simulink model "ExRobotAndEnvironmentControllerContPI"  (Simulink 8.9)
settings: Solver=ode23s  StartTime=0.0  StopTime=1000  FixedStep=.01  RelTol=1e-3  EnableMultiTasking=on
values from neighbouring files (symbols this model uses):
  INITIAL_ROBOT_POS_THETA = 1.5*2    (= 3)    [InitRobotAndEnvironment.m]
  INITIAL_ROBOT_POS_X = 0    [InitRobotAndEnvironment.m]
  INITIAL_ROBOT_POS_Y = 0    [InitRobotAndEnvironment.m]
  INTER_WHEEL_DISTANCE = 0.12    [InitRobotAndEnvironment.m]
  ki_teta = omega*omega/alpha    (= 0.12)    [InitRobotAndEnvironment.m]
  kp_teta = 3*ksi*omega/alpha    (= 0.36)    [InitRobotAndEnvironment.m]
  MAX_SPEED = .5    (= 0.5)    [InitRobotAndEnvironment.m]
  T = 0.002    [InitRobotAndEnvironment.m]
  ts = SENSOR_SAMPLING_TIME    (= 0.001)    [InitRobotAndEnvironment.m]
  ts_anim = ANIMATION_SAMPLING_TIME    (= 0.01)    [InitRobotAndEnvironment.m]
undefined symbols (not defined in the file or in its folder): Env, Robot, RobotInit
settings Model: SuppressorTable=22 serialization::archive 11 0 6 0 0 0 11 0  Creator=alex  LastModifiedBy=dumasart  SnapshotBufferSize=200  SnapshotInterval=50
settings DataIOCC: SignalLoggingSaveFormat=Dataset
settings OptimizationCC: ExpressionDepthLimit=2147483647
settings SFSimCC: SimParseCustomCode=off

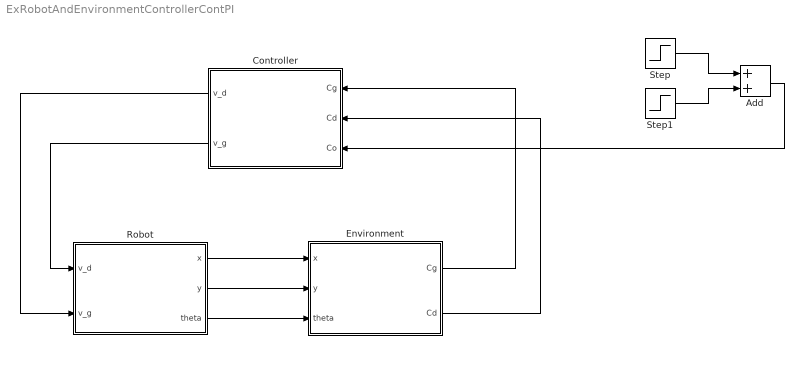
== system ExRobotAndEnvironmentControllerContPI ==
  Add : Sum
  Controller : Subsystem
  Environment : Subsystem
  Robot : Subsystem
  Step : Step  Time=2  Before=50  After=0  SampleTime=1
  Step1 : Step  Time=2.3  After=50  SampleTime=1
  wires:
  Robot/1(x) -> Environment/1(x)
  Robot/2(y) -> Environment/2(y)
  Robot/3(theta) -> Environment/3(theta)
  Environment/1(Cg) -> Controller/1(Cg)
  Environment/2(Cd) -> Controller/2(Cd)
  Controller/1(v_d) -> Robot/2(v_g)
  Controller/2(v_g) -> Robot/1(v_d)
  Step/1 -> Add/1
  Step1/1 -> Add/2
  Add/1 -> Controller/3("Co ")

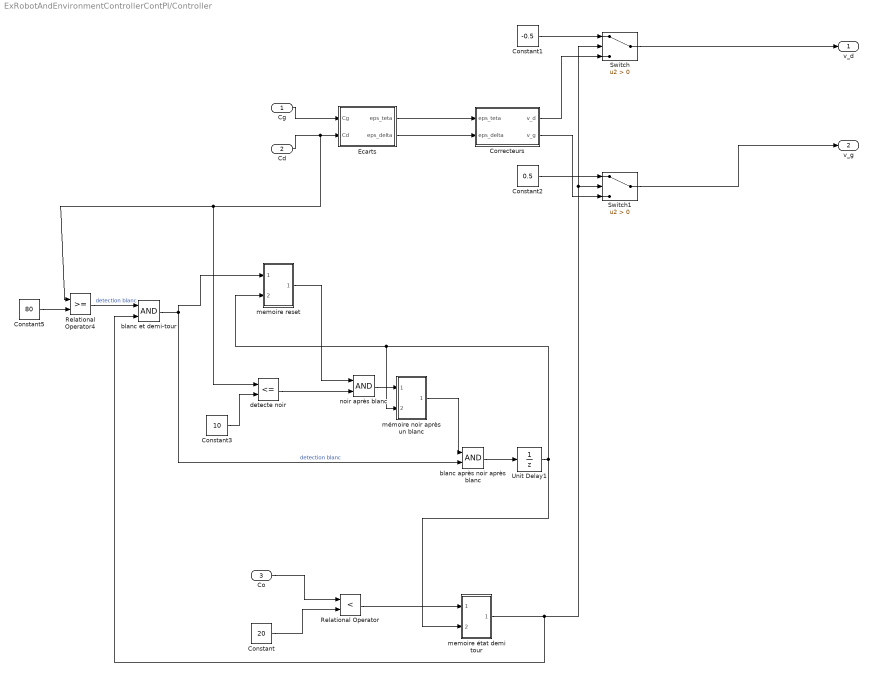
== system ExRobotAndEnvironmentControllerContPI/Controller ==
  Cg : Inport
  Cd : Inport  Port=2
  "Co " : Inport  Port=3  OutDataTypeStr=double
  Constant : Constant  Value=20
  Constant1 : Constant  Value=-0.5
  Constant2 : Constant  Value=0.5
  Constant3 : Constant  Value=10
  Constant5 : Constant  Value=80
  "Correcteurs " : Subsystem
  Ecarts : Subsystem
  Relational Operator : RelationalOperator  Operator=<  OutDataTypeStr=boolean  RndMeth=Simplest
  Relational Operator4 : RelationalOperator  OutDataTypeStr=boolean  RndMeth=Simplest
  Switch : Switch  Criteria=u2 > Threshold
  Switch1 : Switch  Criteria=u2 > Threshold
  Unit Delay1 : UnitDelay  SampleTime=-1
  blanc après noir après blanc : Logic  AllPortsSameDT=off  OutDataTypeStr=boolean
  "blanc et demi-tour " : Logic  AllPortsSameDT=off  OutDataTypeStr=boolean
  "detecte noir " : RelationalOperator  Operator=<=  OutDataTypeStr=boolean  RndMeth=Simplest
  memoire reset : Subsystem
  memoire état demi tour : Subsystem
  mémoire noir après un blanc : Subsystem
  "noir après blanc " : Logic  AllPortsSameDT=off  OutDataTypeStr=boolean
  v_d : Outport
  v_g : Outport  Port=2
  wires:
  Ecarts/2(eps_delta) -> "Correcteurs "/2(eps_delta)
  Cg/1 -> Ecarts/1(Cg)
  Ecarts/1(eps_teta) -> "Correcteurs "/1(eps_teta)
  Constant/1 -> Relational Operator/2
  "Co "/1 -> Relational Operator/1
  Switch/1 -> v_d/1
  Switch1/1 -> v_g/1
  Cd/1 -> "detecte noir "/1, Relational Operator4/1, Ecarts/2(Cd)
  "Correcteurs "/1(v_d) -> Switch/3
  Constant1/1 -> Switch/1
  "Correcteurs "/2(v_g) -> Switch1/3
  Constant2/1 -> Switch1/1
  Constant5/1 -> Relational Operator4/2
  "blanc et demi-tour "/1 -> memoire reset/1(In1), blanc après noir après blanc/2  "detection blanc"
  "detecte noir "/1 -> "noir après blanc "/2
  memoire reset/1(Out1) -> "noir après blanc "/1
  "noir après blanc "/1 -> mémoire noir après un blanc/1(In1)
  mémoire noir après un blanc/1(Out1) -> blanc après noir après blanc/1
  blanc après noir après blanc/1 -> Unit Delay1/1
  memoire état demi tour/1(Out1) -> "blanc et demi-tour "/2, Switch/2, Switch1/2
  Relational Operator/1 -> memoire état demi tour/1(value)
  Constant3/1 -> "detecte noir "/2
  Relational Operator4/1 -> "blanc et demi-tour "/1  "detection blanc"
  Unit Delay1/1 -> memoire état demi tour/2(reset), mémoire noir après un blanc/2(In2), memoire reset/2(In2)

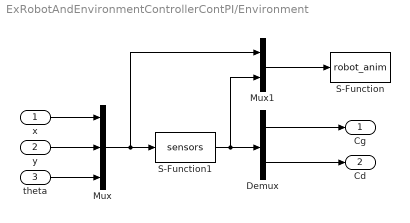
== system ExRobotAndEnvironmentControllerContPI/Environment ==
  x : Inport
  y : Inport  Port=2
  theta : Inport  Port=3
  Demux : Demux  Outputs=2
  Mux : Mux  Inputs=3
  Mux1 : Mux  Inputs=2
  S-Function : S-Function  FunctionName=robot_anim  Parameters=ts_anim,Env,Robot,RobotInit  SFunctionDeploymentMode=off  EnableBusSupport=off
  S-Function1 : S-Function  FunctionName=sensors  Parameters=ts,Env,Robot  SFunctionDeploymentMode=off  EnableBusSupport=off
  Cg : Outport
  Cd : Outport  Port=2
  wires:
  x/1 -> Mux/1
  y/1 -> Mux/2
  theta/1 -> Mux/3
  Mux/1 -> S-Function1/1, Mux1/1
  S-Function1/1 -> Mux1/2, Demux/1
  Mux1/1 -> S-Function/1
  Demux/1 -> Cg/1
  Demux/2 -> Cd/1

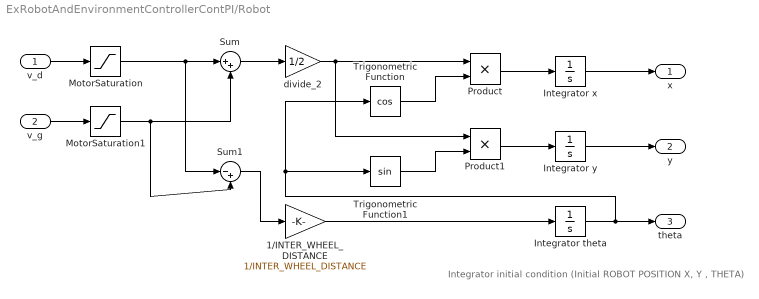
== system ExRobotAndEnvironmentControllerContPI/Robot ==
  note: Integrator initial condition (Initial ROBOT POSITION X, Y , THETA)
  v_d : Inport
  v_g : Inport  Port=2
  1/INTER_WHEEL_DISTANCE : Gain  Gain=1/INTER_WHEEL_DISTANCE
  Integrator theta : Integrator  InitialCondition=INITIAL_ROBOT_POS_THETA
  Integrator x : Integrator  InitialCondition=INITIAL_ROBOT_POS_X
  Integrator y : Integrator  InitialCondition=INITIAL_ROBOT_POS_Y
  MotorSaturation : Saturate  UpperLimit=MAX_SPEED  LowerLimit=-MAX_SPEED
  MotorSaturation1 : Saturate  UpperLimit=MAX_SPEED  LowerLimit=-MAX_SPEED
  Product : Product  RndMeth=Zero
  Product1 : Product  RndMeth=Zero
  Sum : Sum  Inputs=|++
  Sum1 : Sum  Inputs=|-+
  Trigonometric Function : Trigonometry  Operator=cos
  Trigonometric Function1 : Trigonometry
  divide_2 : Gain  Gain=1/2
  x : Outport
  y : Outport  Port=2
  theta : Outport  Port=3
  wires:
  v_d/1 -> MotorSaturation/1
  Integrator x/1 -> x/1
  Integrator y/1 -> y/1
  Integrator theta/1 -> Trigonometric Function/1, Trigonometric Function1/1, theta/1
  Sum/1 -> divide_2/1
  divide_2/1 -> Product1/1, Product/1
  Trigonometric Function/1 -> Product/2
  Trigonometric Function1/1 -> Product1/2
  Product/1 -> Integrator x/1
  Product1/1 -> Integrator y/1
  Sum1/1 -> 1/INTER_WHEEL_DISTANCE/1
  1/INTER_WHEEL_DISTANCE/1 -> Integrator theta/1
  v_g/1 -> MotorSaturation1/1
  MotorSaturation1/1 -> Sum/2, Sum1/2
  MotorSaturation/1 -> Sum/1, Sum1/1

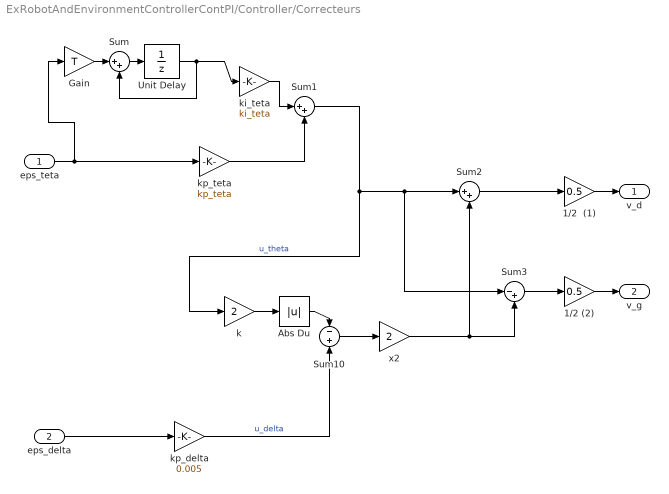
== system ExRobotAndEnvironmentControllerContPI/Controller/Correcteurs  ==
  eps_teta : Inport
  eps_delta : Inport  Port=2
  1/2  (1) : Gain  Gain=0.5  SaturateOnIntegerOverflow=on  OutDataTypeStr=Inherit: Same as input  ParamDataTypeStr=Inherit: Same as input
  1/2 (2) : Gain  Gain=0.5  SaturateOnIntegerOverflow=on  OutDataTypeStr=Inherit: Same as input  ParamDataTypeStr=Inherit: Same as input
  Abs Du : Abs  SaturateOnIntegerOverflow=on
  Gain : Gain  Gain=T
  Sum : Sum  Inputs=|++
  Sum1 : Sum  Inputs=|++  SaturateOnIntegerOverflow=on
  Sum10 : Sum  Inputs=-+  SaturateOnIntegerOverflow=on
  Sum2 : Sum  Inputs=|++  SaturateOnIntegerOverflow=on
  Sum3 : Sum  Inputs=|-+  SaturateOnIntegerOverflow=on
  Unit Delay : UnitDelay  SampleTime=-1
  k : Gain  Gain=2  SaturateOnIntegerOverflow=on  OutDataTypeStr=Inherit: Same as input  ParamDataTypeStr=Inherit: Same as input
  ki_teta : Gain  Gain=ki_teta  SaturateOnIntegerOverflow=on  OutDataTypeStr=Inherit: Same as input  ParamDataTypeStr=Inherit: Same as input
  kp_delta : Gain  Gain=0.005
  kp_teta : Gain  Gain=kp_teta  SaturateOnIntegerOverflow=on  OutDataTypeStr=Inherit: Same as input  ParamDataTypeStr=Inherit: Same as input
  x2 : Gain  Gain=2  SaturateOnIntegerOverflow=on  OutDataTypeStr=Inherit: Same as input  ParamDataTypeStr=Inherit: Same as input
  v_d : Outport
  v_g : Outport  Port=2
  wires:
  ki_teta/1 -> Sum1/1
  kp_teta/1 -> Sum1/2
  Sum2/1 -> 1/2  (1)/1
  Sum3/1 -> 1/2 (2)/1
  k/1 -> Abs Du/1
  kp_delta/1 -> Sum10/2  "u_delta"
  Abs Du/1 -> Sum10/1
  x2/1 -> Sum2/2, Sum3/2
  Sum10/1 -> x2/1
  Sum1/1 -> k/1, Sum2/1, Sum3/1  "u_theta"
  1/2  (1)/1 -> v_d/1
  1/2 (2)/1 -> v_g/1
  eps_delta/1 -> kp_delta/1
  eps_teta/1 -> Gain/1, kp_teta/1
  Gain/1 -> Sum/1
  Sum/1 -> Unit Delay/1
  Unit Delay/1 -> Sum/2, ki_teta/1

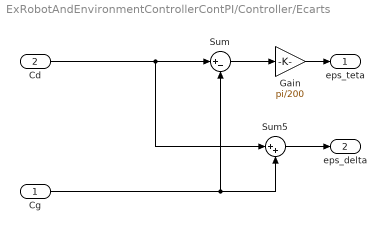
== system ExRobotAndEnvironmentControllerContPI/Controller/Ecarts ==
  Cg : Inport
  Cd : Inport  Port=2
  Gain : Gain  Gain=pi/200
  Sum : Sum  Inputs=|+-
  Sum5 : Sum  Inputs=|++
  eps_teta : Outport
  eps_delta : Outport  Port=2
  wires:
  Sum/1 -> Gain/1
  Cd/1 -> Sum/1, Sum5/1
  Cg/1 -> Sum/2, Sum5/2
  Gain/1 -> eps_teta/1
  Sum5/1 -> eps_delta/1

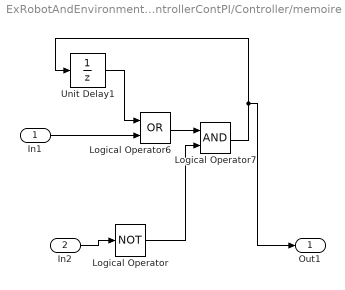
== system ExRobotAndEnvironmentControllerContPI/Controller/memoire reset ==
  In1 : Inport
  In2 : Inport  Port=2
  Logical Operator : Logic  Operator=NOT  AllPortsSameDT=off  OutDataTypeStr=boolean
  Logical Operator6 : Logic  Operator=OR  AllPortsSameDT=off  OutDataTypeStr=boolean
  Logical Operator7 : Logic  AllPortsSameDT=off  OutDataTypeStr=boolean
  Unit Delay1 : UnitDelay  SampleTime=-1
  Out1 : Outport
  wires:
  Logical Operator7/1 -> Unit Delay1/1, Out1/1
  In1/1 -> Logical Operator6/2
  Unit Delay1/1 -> Logical Operator6/1
  Logical Operator6/1 -> Logical Operator7/1
  Logical Operator/1 -> Logical Operator7/2
  In2/1 -> Logical Operator/1

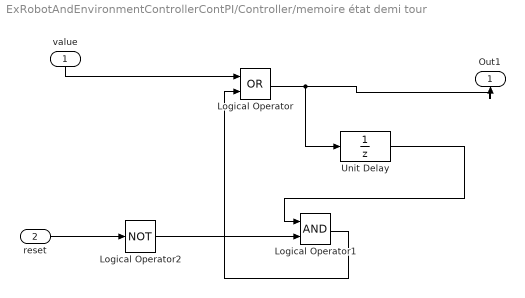
== system ExRobotAndEnvironmentControllerContPI/Controller/memoire état demi tour ==
  value : Inport
  reset : Inport  Port=2
  Logical Operator : Logic  Operator=OR  AllPortsSameDT=off  OutDataTypeStr=boolean
  Logical Operator1 : Logic  AllPortsSameDT=off  OutDataTypeStr=boolean
  Logical Operator2 : Logic  Operator=NOT  AllPortsSameDT=off  OutDataTypeStr=boolean
  Unit Delay : UnitDelay  SampleTime=-1
  Out1 : Outport
  wires:
  Logical Operator2/1 -> Logical Operator1/2
  Logical Operator/1 -> Unit Delay/1, Out1/1
  reset/1 -> Logical Operator2/1
  value/1 -> Logical Operator/1
  Logical Operator1/1 -> Logical Operator/2
  Unit Delay/1 -> Logical Operator1/1

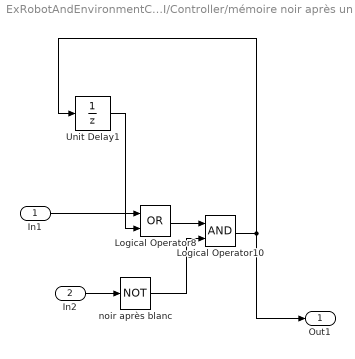
== system ExRobotAndEnvironmentControllerContPI/Controller/mémoire noir après un blanc ==
  In1 : Inport
  In2 : Inport  Port=2
  Logical Operator10 : Logic  AllPortsSameDT=off  OutDataTypeStr=boolean
  Logical Operator8 : Logic  Operator=OR  AllPortsSameDT=off  OutDataTypeStr=boolean
  Unit Delay1 : UnitDelay  SampleTime=-1
  "noir après blanc " : Logic  Operator=NOT  AllPortsSameDT=off  OutDataTypeStr=boolean
  Out1 : Outport
  wires:
  In1/1 -> Logical Operator8/1
  Logical Operator8/1 -> Logical Operator10/1
  Logical Operator10/1 -> Unit Delay1/1, Out1/1
  Unit Delay1/1 -> Logical Operator8/2
  In2/1 -> "noir après blanc "/1
  "noir après blanc "/1 -> Logical Operator10/2
